simulink model "preLookupTestGen14"  (R2017b)
settings: Solver=FixedStepDiscrete  StartTime=0.0  StopTime=10.0  RelTol=1e-3
undefined symbols (not defined in the file): Block_TestLib, trigger
settings Model: Creator=ktrinh  LastModifiedBy=ktrinh
settings DebuggingCC: ParameterOverflowMsg=none

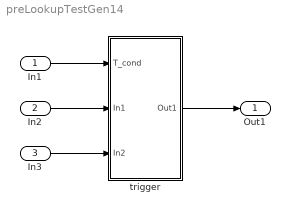
== system preLookupTestGen14 ==
  In1 : Inport
  In2 : Inport  Port=2
  In3 : Inport  Port=3
  trigger : Subsystem  AncestorBlock=Block_TestLib/trigger
  Out1 : Outport
  wires:
  In1/1 -> trigger/1(T_cond)
  In2/1 -> trigger/2(In1)
  In3/1 -> trigger/3(In2)
  trigger/1(Out1) -> Out1/1

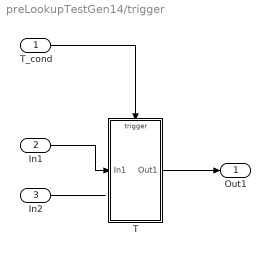
== system preLookupTestGen14/trigger ==
  T_cond : Inport  OutDataTypeStr=boolean
  In1 : Inport  Port=2
  In2 : Inport  Port=3
  T : Subsystem  TreatAsAtomicUnit=on
  Out1 : Outport
  wires:
  T_cond/1 -> T/Trigger
  In1/1 -> T/1(In1)
  In2/1 -> ?
  T/1(Out1) -> Out1/1

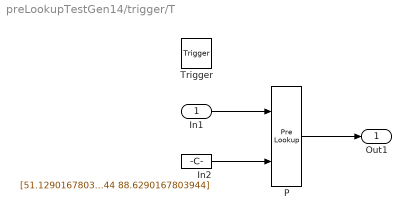
== system preLookupTestGen14/trigger/T ==
  In1 : Inport  OutDataTypeStr=double  PortDimensions=[2,3]
  Trigger : TriggerPort  VariantControl=Variant
  In2 : Constant  Value=[51.1290167803944 52.6290167803944 54.1290167803944 55.6290167803944 57.1290167803944 58.6290167803944 60.1290167803944 61.6290167803944 63.1290167803944 64.6290167803944 66.1290167803944 67.6290167803944 69.1290167803944 70.6290167803944 72.1290167803944 73.6290167803944 75.1290167803944 76.6290167803944 78.1290167803944 79.6290167803944 81.1290167803944 82.6290167803944 84.1290167803944 85.6290167803944 87.1290167803944 88.6290167803944]
  P : PreLookup  BreakpointsDataSource=Input port  BreakpointsData=[10:10:110]  OutputSelection=Index only  IndexSearchMethod=Linear search  BeginIndexSearchUsingPreviousIndexResult=on  BreakpointDataTypeStr=int8  IndexDataTypeStr=int16  FractionDataTypeStr=double  RndMeth=Ceiling
      settings: InputPortMap=u0,p1
  Out1 : Outport
  wires:
  In1/1 -> P/1
  In2/1 -> P/2
  P/1 -> Out1/1
